simulink model "controller_dev_sg_RCP"  (R2018b)
settings: configuration reference "Active" (kept outside this file)
model workspace (MAT data in the model file):
  m = 1000
undefined symbols (not defined in the file or in its folder): C, tS, TUMHealthStatus, TUMVehicleState
libraries: xpcrtudplib x6, simulink x6, canmsglib x6, etargetslib x5, misc x4, speedgoatlib_IO614 x3, slrtlib x2
(part 1 of 3)
settings Model: DataDictionary=controller_dev_sg.sldd  sg_rtwmakecfg_data=_sglibc__IO61X_Library_  PauseTimes=9.280  Creator=wischnewski  LastModifiedBy=ge34qer

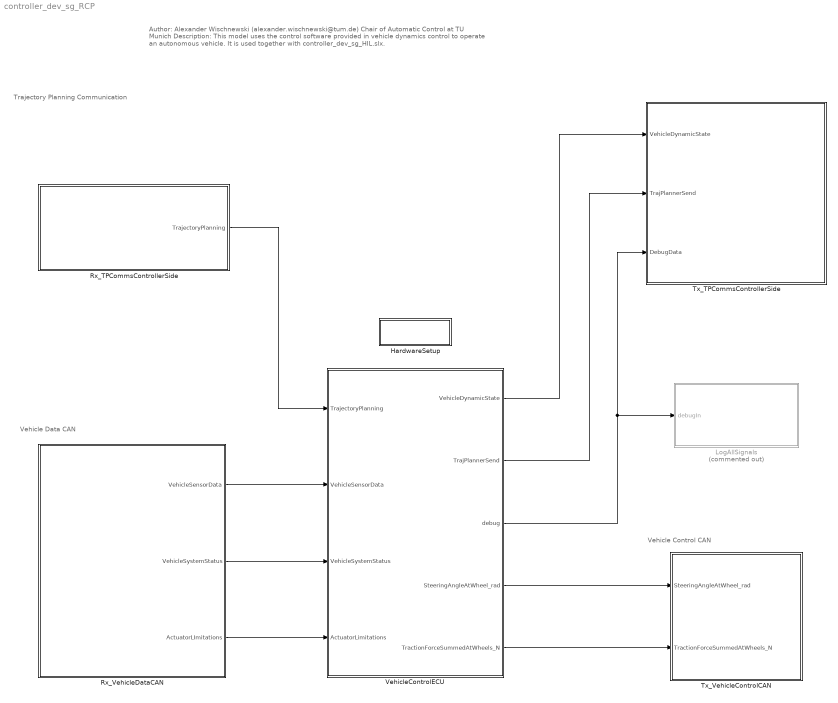
== system controller_dev_sg_RCP ==
  note: Trajectory Planning Communication
  note: Vehicle Control CAN
  note: Vehicle Data CAN
  note: Author: Alexander Wischnewski (alexander.wischnewski@tum.de)
      | Chair of Automatic Control at TU Munich
      |
      | Description: This model uses the control software provided in vehicle dynamics control to operate an autonomous vehicle.
      | It is used together with controller_dev_sg_HIL.slx.
  HardwareSetup : Subsystem
  LogAllSignals : Subsystem  Commented=on
  Rx_TPCommsControllerSide : Subsystem
  Rx_VehicleDataCAN : Subsystem
  Tx_TPCommsControllerSide : Subsystem
  Tx_VehicleControlCAN : Subsystem
  VehicleControlECU : Subsystem
  wires:
  VehicleControlECU/3(debug) -> Tx_TPCommsControllerSide/3(DebugData), LogAllSignals/1(debugIn)
  Rx_TPCommsControllerSide/1(TrajectoryPlanning) -> VehicleControlECU/1(TrajectoryPlanning)
  VehicleControlECU/1(VehicleDynamicState) -> Tx_TPCommsControllerSide/1(VehicleDynamicState)
  VehicleControlECU/2(TrajPlannerSend) -> Tx_TPCommsControllerSide/2(TrajPlannerSend)
  Rx_VehicleDataCAN/3(ActuatorLImitations) -> VehicleControlECU/4(ActuatorLimitations)
  Rx_VehicleDataCAN/2(VehicleSystemStatus) -> VehicleControlECU/3(VehicleSystemStatus)
  Rx_VehicleDataCAN/1(VehicleSensorData) -> VehicleControlECU/2(VehicleSensorData)
  VehicleControlECU/4(SteeringAngleAtWheel_rad) -> Tx_VehicleControlCAN/1(SteeringAngleAtWheel_rad)
  VehicleControlECU/5(TractionForceSummedAtWheels_N) -> Tx_VehicleControlCAN/2(TractionForceSummedAtWheels_N)

== system controller_dev_sg_RCP/HardwareSetup ==
  CAN & LIN Setup : speedgoatlib_IO614/CAN & LIN Setup  id=1  drLtr=C:  PCISlot=-1  port1=CAN (HS/LS)  port2=CAN (HS)  port3=Disable  port4=Disable  opModeCAN1=Highspeed (HS)  bdrCAN1=1 MBaud  usrBdrCAN1=[5, 1, 13, 2]  stdAccMaskCAN1=[0, 0]  extAccMaskCAN1=[0, 0]  opModeCAN2=Highspeed (HS)  bdrCAN2=1 MBaud  usrBdrCAN2=[5, 1, 13, 2]  stdAccMaskCAN2=[0, 0]  extAccMaskCAN2=[0, 0]  opModeCAN3=Highspeed (HS)  bdrCAN3=1 MBaud  usrBdrCAN3=[5, 1, 13, 2]  stdAccMaskCAN3=[0, 0]  extAccMaskCAN3=[0, 0]  opModeCAN4=Highspeed (HS)  bdrCAN4=1 MBaud  usrBdrCAN4=[5, 1, 13, 2]  stdAccMaskCAN4=[0, 0]  extAccMaskCAN4=[0, 0]  initStruct=[]  termStruct=[]  opModeLIN=Master  bdrLIN=19200  protl=IO614  qtyMod=1  chNo=[1, 2, 3, 4]  ptTypes=[1, 1, 1, 1, 2]  protlHelpIdx=[0, 1, 2, 3, 0]  isFDMod=0  drvLtr=C:  opModeLIN2=Master  bdrLIN2=19200
      settings: SourceProductName=Simulink Real-Time: Speedgoat Library
  "Real-time UDP Configuration " : xpcrtudplib/UDP Configure  Priority=1  IpAddress=10.0.0.1  SubnetMask=255.255.255.0  Gateway=0.0.0.0  PciBus=14  PciSlot=0  PciFunction=0  ID=3  tune=0  disable=off  enableMulticast=off  MulticastIpAddress={}  MulticastMask={}
      settings: SourceProductName=Simulink Real-Time  SourceProductBaseCode=XP
